simulink model "dbdc_ut"  (Simulink 8.1)
settings: Solver=FixedStepDiscrete  StartTime=0.0  StopTime=Inf  FixedStep=0.005  RelTol=1e-3
PostLoadFcn:
  | , if any(exist('dsrtsu_mdlpostloadfcn', 'file') == [2, 3, 6]), try dsrtsu_mdlpostloadfcn('Execute', bdroot); catch fprintf('Error in PostLoadFcn (dsrtsu_mdlpostloadfcn) for model "%s":\n %s\n', bdroot, lasterr); end, end,
undefined symbols (not defined in the file or in its folder): KJUD_FCWActiveDriverDelay_ms, KJUD_FCWAggrDriverDelay_ms, ZERO_FLOAT
libraries: siltestlib x3
settings Model: DSRTSU_INTERNAL_RTI_VER=450  DSRTSU_INTERNAL_RTI_TYPE=rti1401  RTICANMMDATA=struct('GeneralSetupData',struct('modelroot','D:\ELN150201_TAIWAN\trunk\AdasDragon\software\sw_development\arch\app\jud','generalsettings',struct('filesettings',struct('destfolder',struct('Name','RTICANMM_FILES','Check',1),'buildfolder',struct('Name','.','Check',1),'AbsDestfolder',struct('Name','D:\ELN150201_TAIWAN\trunk\AdasDragon\software\sw_development\arch\app\jud\RTICANMM_FILES'),'AbsBuildfolder',struct('Name','D:\ELN150201_TAIWAN\trunk\AdasDragon\software\sw_development\arch\app\jud'))),'options',struct('addpaths',1,'rmpaths',1,'addtrcexclusion',logical(1),'cannavigator',struct('checkmonitoring',0),'show_usrtrc',0,'use_usrtrc',0),'advanced',struct('options',[1 1 1 1 1 1 1 1 1 1 1 1 1 1 1 1 1 1 1 1 1 1 1 1 1 1 1 1 1 1 1 1 1 1 1 1 1 1 1 1 1 1 1 1 1 1 1 1 1 1 1 1 1 1 1 1 1 1 1 1 1 1 1 1 1 1 1 1 1 1 1 1 1 1 1 1 1 1 1 1 1 1 1 1 1 1 1 1 1 1 1 1 1 1 1 1 1 1 1 1]),'MPSetup',{{}},'modelname','dbdc_ut','block','dbdc_ut'))  DSRTSU_INTERNAL_RTIFPGA=40  Creator=idiada  LastModifiedBy=AT015555  BufferReuse=off
settings DataIOCC: SignalLoggingSaveFormat=Dataset
settings OptimizationCC: BlockReduction=off  OptimizeBlockIOStorage=off  BufferReuse=off  ExpressionFolding=off  ExpressionDepthLimit=128  LocalBlockOutputs=off
settings DebuggingCC: FcnCallInpInsideContextMsg=EnableAllAsError
settings HardwareCC: TargetHWDeviceType=Generic->Custom
settings RTWCC: SystemTargetFile=rti1401.tlc  MakeCommand=make_rti  TemplateMakefile=rti1401.tmf  Description=dSPACE DS1401 Hardware Platform  ProcessScript=rti1401_make_rtw_hook
settings STFCustomTargetCC: CodeReplacementLibrary=ANSI_C  ParMdlRefBuildCompliant=on  GeneratePreprocessorConditionals=Disable all  MatFileLogging=on  SystemTargetFile=rti1401.tlc
settings GRTTargetCC: CompOptLevelCompliant=off  ConcurrentExecutionCompliant=off  ExtModeMexFile=noextcomm
settings CustomProperty: DataType=RTWOptions_EnumType_C__Program Files (x86)_dSPACE RCPHIL 2014-B_MATLAB_RTI_RTI1401_TLC_rti1401_1InitialSimState  Value=RUN
settings EnumStrPairs: String=RUN

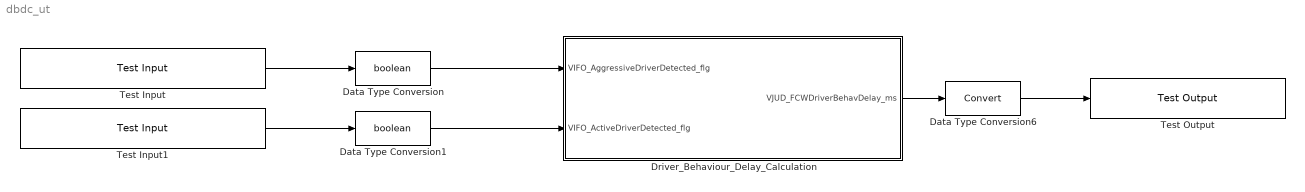
== system dbdc_ut ==
  Data Type Conversion : DataTypeConversion  OutDataTypeStr=boolean
  Data Type Conversion1 : DataTypeConversion  OutDataTypeStr=boolean
  Data Type Conversion6 : DataTypeConversion
  Driver_Behaviour_Delay_Calculation : Subsystem
  Test Input : siltestlib/Test Input  varname=VIFO_AggressiveDriverDetected_flg  sampletime=0.005
  Test Input1 : siltestlib/Test Input  varname=VIFO_ActiveDriverDetected_flg  sampletime=0.005
  Test Output : siltestlib/Test Output  varname=VJUD_FCWDriverBehavDelay_ms  sampletime=-1
  wires:
  Test Input/1 -> Data Type Conversion/1
  Data Type Conversion/1 -> Driver_Behaviour_Delay_Calculation/1(VIFO_AggressiveDriverDetected_flg)
  Test Input1/1 -> Data Type Conversion1/1
  Data Type Conversion1/1 -> Driver_Behaviour_Delay_Calculation/2(VIFO_ActiveDriverDetected_flg)
  Driver_Behaviour_Delay_Calculation/1(VJUD_FCWDriverBehavDelay_ms) -> Data Type Conversion6/1
  Data Type Conversion6/1 -> Test Output/1

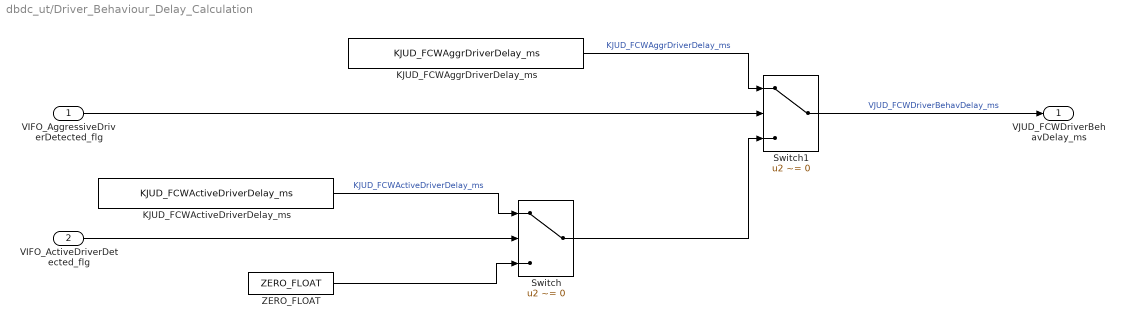
== system dbdc_ut/Driver_Behaviour_Delay_Calculation ==
  VIFO_AggressiveDriverDetected_flg : Inport
  VIFO_ActiveDriverDetected_flg : Inport  Port=2
  KJUD_FCWActiveDriverDelay_ms : Constant  Value=KJUD_FCWActiveDriverDelay_ms  OutDataTypeStr=single
  KJUD_FCWAggrDriverDelay_ms : Constant  Value=KJUD_FCWAggrDriverDelay_ms  OutDataTypeStr=single
  Switch : Switch  Criteria=u2 ~= 0
  Switch1 : Switch  Criteria=u2 ~= 0
  ZERO_FLOAT : Constant  Value=ZERO_FLOAT  OutDataTypeStr=single
  VJUD_FCWDriverBehavDelay_ms : Outport
  wires:
  VIFO_ActiveDriverDetected_flg/1 -> Switch/2
  Switch1/1 -> VJUD_FCWDriverBehavDelay_ms/1  "VJUD_FCWDriverBehavDelay_ms"
  ZERO_FLOAT/1 -> Switch/3
  KJUD_FCWActiveDriverDelay_ms/1 -> Switch/1  "KJUD_FCWActiveDriverDelay_ms"
  VIFO_AggressiveDriverDetected_flg/1 -> Switch1/2
  Switch/1 -> Switch1/3
  KJUD_FCWAggrDriverDelay_ms/1 -> Switch1/1  "KJUD_FCWAggrDriverDelay_ms"
